simulink model "qrotor_sim"  (R2023a)
settings: Solver=VariableStepAuto  StartTime=0.0  StopTime=10.0  RelTol=1e-3
values from neighbouring files (symbols this model uses):
  x0 = [ ... (first row only)    [sim_start.m]
undefined symbols (not defined in the file or in its folder): qrotor_model
settings Model: Creator=stoyanov  LastModifiedBy=stoyanov

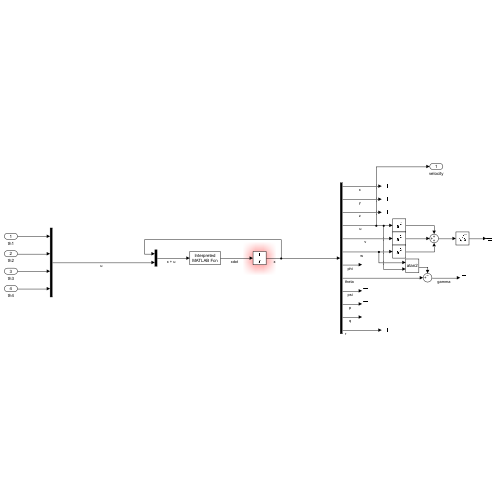
[thumbnail: Simulink's stored preview of the top-level diagram]
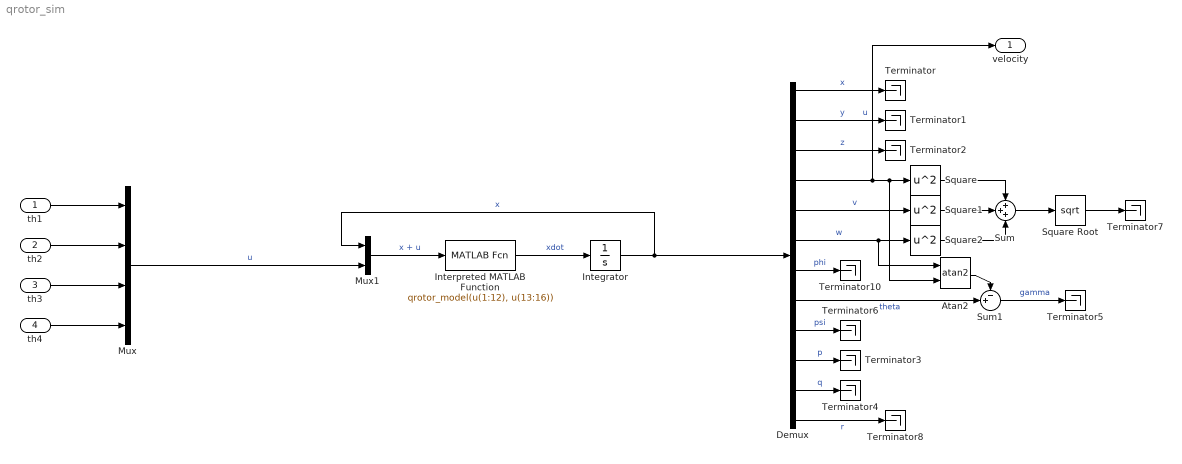
== system qrotor_sim ==
  th1 : Inport  PortDimensions=1
  th2 : Inport  Port=2  PortDimensions=1
  th3 : Inport  Port=3  PortDimensions=1
  th4 : Inport  Port=4  PortDimensions=1
  Atan2 : Trigonometry  Operator=atan2
  Demux : Demux  Outputs=12
  Integrator : Integrator  InitialCondition=x0
  Interpreted MATLAB Function : MATLABFcn  MATLABFcn=qrotor_model(u(1:12), u(13:16))  OutputDimensions=12
  Mux : Mux
  Mux1 : Mux  Inputs=2
  Square : Math  Operator=square
  Square Root : Sqrt
  Square1 : Math  Operator=square
  Square2 : Math  Operator=square
  Sum : Sum  Inputs=+++
  Sum1 : Sum  Inputs=-+|
  Terminator{,1..8,10} (10 alike) : Terminator
  velocity : Outport
  wires:
  th1/1 -> Mux/1
  th2/1 -> Mux/2
  th3/1 -> Mux/3
  th4/1 -> Mux/4
  Mux1/1 -> Interpreted MATLAB Function/1  "x + u"
  Mux/1 -> Mux1/2  "u"
  Interpreted MATLAB Function/1 -> Integrator/1  "xdot"
  Integrator/1 -> Mux1/1, Demux/1  "x"
  Demux/1 -> Terminator/1  "x"
  Demux/2 -> Terminator1/1  "y"
  Demux/3 -> Terminator2/1  "z"
  Demux/4 -> velocity/1, Atan2/2, Square/1  "u"
  Demux/5 -> Square1/1  "v"
  Demux/6 -> Atan2/1, Square2/1  "w"
  Square1/1 -> Sum/2
  Square/1 -> Sum/1
  Square2/1 -> Sum/3
  Sum/1 -> Square Root/1
  Square Root/1 -> Terminator7/1
  Demux/10 -> Terminator3/1  "p"
  Demux/11 -> Terminator4/1  "q"
  Demux/12 -> Terminator8/1  "r"
  Demux/7 -> Terminator10/1  "phi"
  Demux/8 -> Sum1/2  "theta"
  Demux/9 -> Terminator6/1  "psi"
  Atan2/1 -> Sum1/1
  Sum1/1 -> Terminator5/1  "gamma"
